simulink model "vehicle3dof"  (R2023a)
settings: Solver=FixedStepAuto  StartTime=0.0  StopTime=50  FixedStep=0.01  RelTol=1e-3
model workspace (MAT data in the model file):
  Cy_f1 = 128915.5
  Cy_r1 = 85943.6
  Izz1 = 1536.7
  a1 = 1.015
  a_max = Simulink.Parameter
  a_max.Value = [1.5 9000 9000]
  a_max.DataType = 'auto'
  a_max.Complexity = 'real'
  a_max.Dimensions = [1 3]
  a_min = Simulink.Parameter
  a_min.Value = [-1.5 -9000 -9000]
  a_min.DataType = 'auto'
  a_min.Complexity = 'real'
  a_min.Dimensions = [1 3]
  adva_max = Simulink.Parameter
  adva_max.Value = [0.05 300 300]
  adva_max.DataType = 'auto'
  adva_max.Complexity = 'real'
  adva_max.Dimensions = [1 3]
  adva_min = Simulink.Parameter
  adva_min.Value = [-0.05 -300 -300]
  adva_min.DataType = 'auto'
  adva_min.Complexity = 'real'
  adva_min.Dimensions = [1 3]
  b1 = 1.895
  done_range = Simulink.Parameter
  done_range.Value = [6 5 0.523598775598]
  done_range.DataType = 'double'
  done_range.Complexity = 'real'
  done_range.Dimensions = [1 3]
  h1 = 0.54
  noise_seed = Simulink.Parameter
  noise_seed.Value = 23341
  noise_seed.DataType = 'auto'
  noise_seed.Complexity = 'real'
  noise_seed.Dimensions = [1 1]
  punish_Q = Simulink.Parameter
  punish_Q.Value = [1 1 10 0.5]
  punish_Q.DataType = 'auto'
  punish_Q.Complexity = 'real'
  punish_Q.Dimensions = [1 4]
  punish_R = Simulink.Parameter
  punish_R.Value = [5 1e-06 1e-06]
  punish_R.DataType = 'auto'
  punish_R.Complexity = 'real'
  punish_R.Dimensions = [1 3]
  ref_A = Simulink.Parameter
  ref_A.Value = [0.3 0.8 1.5]
  ref_A.DataType = 'auto'
  ref_A.Complexity = 'real'
  ref_A.Dimensions = [1 3]
  ref_T = Simulink.Parameter
  ref_T.Value = [100 200 400]
  ref_T.DataType = 'auto'
  ref_T.Complexity = 'real'
  ref_T.Dimensions = [1 3]
  ref_V = Simulink.Parameter
  ref_V.Value = 20
  ref_V.DataType = 'auto'
  ref_V.Complexity = 'real'
  ref_V.Dimensions = [1 1]
  ref_fai = Simulink.Parameter
  ref_fai.Value = [0 0.523598775598 1.0471975512]
  ref_fai.DataType = 'auto'
  ref_fai.Complexity = 'real'
  ref_fai.Dimensions = [1 3]
  sigma_f1 = 0.1
  sigma_r1 = 0.1
  x_ini = Simulink.Parameter
  x_ini.Value = [0 0 20 0 0 0]
  x_ini.DataType = 'auto'
  x_ini.Complexity = 'real'
  x_ini.Dimensions = [1 6]
  x_max = Simulink.Parameter
  x_max.Value = [9999 9999 9999 9999 9999 9999]
  x_max.DataType = 'auto'
  x_max.Complexity = 'real'
  x_max.Dimensions = [1 6]
  x_min = Simulink.Parameter
  x_min.Value = [-9999 -9999 -9999 -9999 -9999 -9999]
  x_min.DataType = 'auto'
  x_min.Complexity = 'real'
  x_min.Dimensions = [1 6]
libraries: autolibshared x1, simulink x1
settings Model: TunableVars=a_max,a_min,adva_max,adva_min,x_ini,x_max,x_min  TunableVarsStorageClass=Auto,Auto,Auto,Auto,Auto,Auto,Auto  TunableVarsTypeQualifier=,,,,,,  ParameterArgumentNames=a_max,a_min,adva_max,adva_min,done_range,noise_seed,punish_Q,punish_R,ref_A,ref_T,ref_V,ref_fai,x_ini,x_max,x_min  Creator=hjzsj  LastModifiedBy=Asus
settings ConfigSet: Description=Config for code generation python binding.
settings SolverCC: AlgebraicLoopSolver=TrustRegion
settings OptimizationCC: DefaultParameterBehavior=Inlined  UseDivisionForNetSlopeComputation=on  UseFloatMulNetSlope=on  StrengthReduction=on  PassReuseOutputArgsAs=Individual arguments  ZeroExternalMemoryAtStartup=off  ZeroInternalMemoryAtStartup=off  NoFixptDivByZeroProtection=on  EfficientFloat2IntCast=on  OptimizeBlockOrder=speed  OptimizationPriority=Speed  OptimizationCustomize=off  MultiThreadedLoops=on  EfficientTunableParamExpr=on
settings DebuggingCC: ParameterTunabilityLossMsg=error  UnconnectedInputMsg=warning  UnconnectedOutputMsg=warning  UnconnectedLineMsg=warning  ArithmeticOperatorsInVariantConditions=warning
settings HardwareCC: ProdLongLongMode=on  TargetPreprocMaxBitsSint=64  TargetPreprocMaxBitsUint=64
settings ModelReferenceCC: EnableRefExpFcnMdlSchedulingChecks=on
settings SFSimCC: MATLABDynamicMemAlloc=off  CustomCodeUndefinedFunction=UseInterfaceOnly  SimTargetLang=C++
settings RTWCC: Description=Embedded Coder  SystemTargetFile=ert.tlc  GenCodeOnly=on  TemplateMakefile=ert_default_tmf  PostCodeGenCommand=slxpy.postprocess(modelName,buildInfo)  RetainRTWFile=on  PortableWordSizes=on  TargetLang=C++  DLArmComputeVersion=19.05
settings CodeAppCC: ForceParamTrailComments=on  CommentStyle=Multi-line  IgnoreCustomStorageClasses=off  MaxIdLength=64  OperatorAnnotations=on  SimulinkDataObjDesc=on  SFDataObjDesc=on  MATLABFcnDesc=on  MangleLength=4  InsertBlockDesc=on  StateflowObjectComments=on  MATLABSourceComments=on
settings ERTTargetCC: TargetLangStandard=C++11 (ISO)  SupportAbsoluteTime=off  CodeInterfacePackaging=C++ class  SupportComplex=off  SupportContinuousTime=on  SupportVariableSizeSignals=on  InlinedParameterPlacement=NonHierarchical  RootIOFormat=Structure reference  ERTCustomFileTemplate=example_file_process.tlc

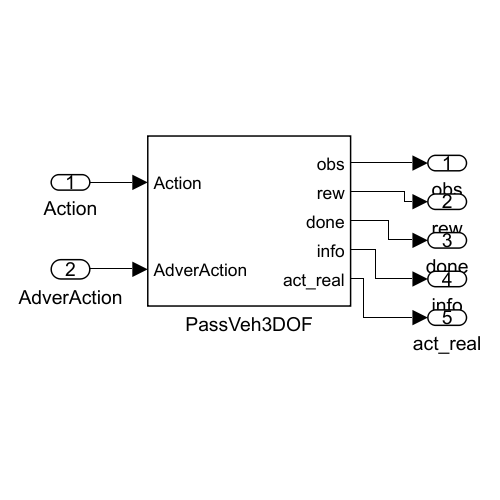
[thumbnail: Simulink's stored preview of the top-level diagram]
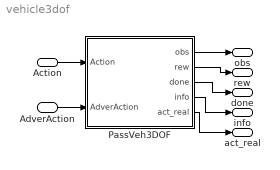
== system vehicle3dof ==
  Action : Inport  PortDimensions=3
  AdverAction : Inport  Port=2
  "PassVeh3DOF " : Subsystem
  obs : Outport
  rew : Outport  Port=2
  done : Outport  Port=3
  info : Outport  Port=4
  act_real : Outport  Port=5
  wires:
  "PassVeh3DOF "/1(obs) -> obs/1
  "PassVeh3DOF "/2(rew) -> rew/1
  Action/1 -> "PassVeh3DOF "/1(Action)
  AdverAction/1 -> "PassVeh3DOF "/2(AdverAction)
  "PassVeh3DOF "/3(done) -> done/1
  "PassVeh3DOF "/4(info) -> info/1
  "PassVeh3DOF "/5(act_real) -> act_real/1

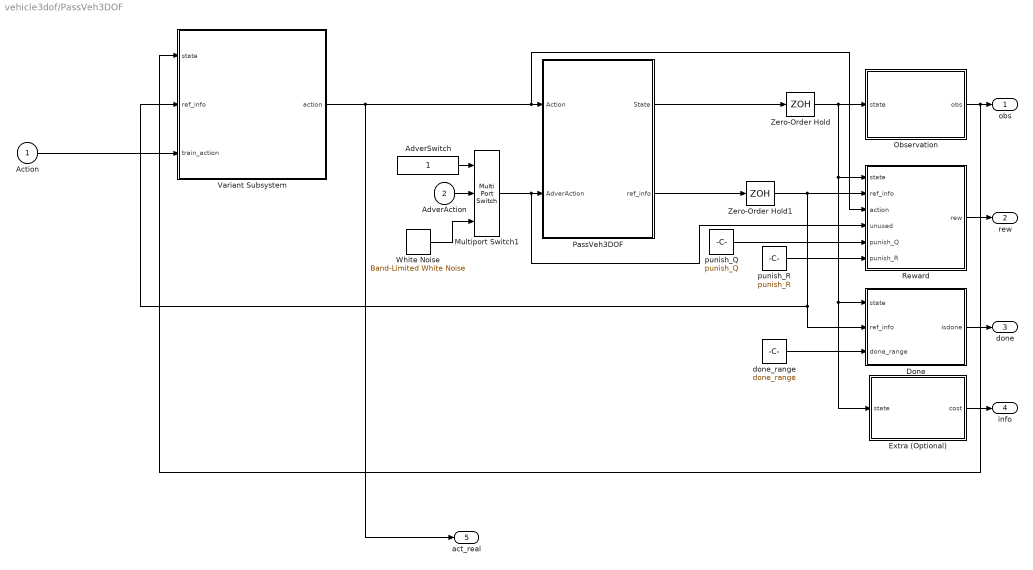
== system vehicle3dof/PassVeh3DOF  ==
  Action : Inport
  AdverAction : Inport  Port=2
  AdverSwitch : Constant
  Done : MATLAB Function  TreatAsAtomicUnit=on
  Extra (Optional) : MATLAB Function  TreatAsAtomicUnit=on
  Multiport Switch1 : MultiPortSwitch  Inputs=2  SaturateOnIntegerOverflow=off  InputSameDT=off
  Observation : MATLAB Function  TreatAsAtomicUnit=on
  "PassVeh3DOF " : Subsystem
  Reward : MATLAB Function  TreatAsAtomicUnit=on
  Variant Subsystem : Subsystem  Variant=on  VariantControlMode=label  LabelModeActiveChoice=Train
  White Noise : simulink/Sources/Band-Limited White Noise  Cov=[0.5, 100, 100]  Ts=0.02  seed=noise_seed
  Zero-Order Hold : ZeroOrderHold  SampleTime=-1
  Zero-Order Hold1 : ZeroOrderHold  SampleTime=-1
  done_range : Constant  Value=done_range
  punish_Q : Constant  Value=punish_Q
  punish_R : Constant  Value=punish_R
  obs : Outport
  rew : Outport  Port=2
  done : Outport  Port=3
  info : Outport  Port=4
  act_real : Outport  Port=5
  wires:
  Action/1 -> Variant Subsystem/3(train_action)
  Multiport Switch1/1 -> Reward/4(unused), "PassVeh3DOF "/2(AdverAction)
  AdverSwitch/1 -> Multiport Switch1/1
  White Noise/1 -> Multiport Switch1/3
  AdverAction/1 -> Multiport Switch1/2
  Zero-Order Hold/1 -> Extra (Optional)/1(state), Done/1(state), Reward/1(state), Observation/1(state)
  "PassVeh3DOF "/1(State) -> Zero-Order Hold/1
  Observation/1(obs) -> Variant Subsystem/1(state), obs/1
  Reward/1(rew) -> rew/1
  Extra (Optional)/1(cost) -> info/1
  "PassVeh3DOF "/2(ref_info) -> Zero-Order Hold1/1
  punish_Q/1 -> Reward/5(punish_Q)
  punish_R/1 -> Reward/6(punish_R)
  done_range/1 -> Done/3(done_range)
  Done/1(isdone) -> done/1
  Zero-Order Hold1/1 -> Done/2(ref_info), Variant Subsystem/2(ref_info), Reward/2(ref_info)
  Variant Subsystem/1(action) -> Reward/3(action), "PassVeh3DOF "/1("Action "), act_real/1

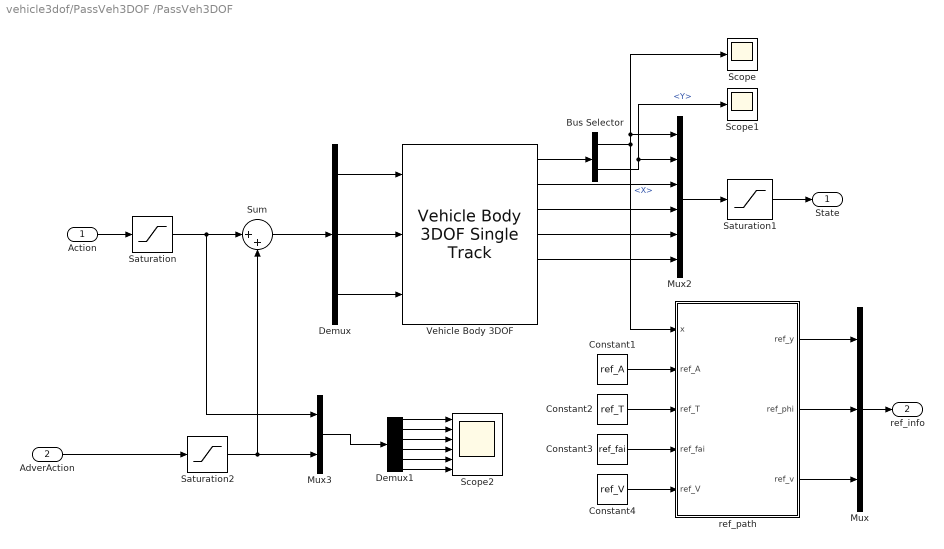
== system vehicle3dof/PassVeh3DOF /PassVeh3DOF  ==
  "Action " : Inport
  AdverAction : Inport  Port=2
  " ref_path " : MATLAB Function  TreatAsAtomicUnit=on
  Bus Selector : BusSelector  OutputSignals=InertFrm.Cg.Disp.X,InertFrm.Cg.Disp.Y
  Constant1 : Constant  Value=ref_A
  Constant2 : Constant  Value=ref_T
  Constant3 : Constant  Value=ref_fai
  Constant4 : Constant  Value=ref_V
  Demux : Demux  Outputs=3
  Demux1 : Demux  Outputs=6
  Mux : Mux  Inputs=3
  Mux2 : Mux  Inputs=6
  Mux3 : Mux  Inputs=2
  Saturation : Saturate  UpperLimit=a_max  LowerLimit=a_min
  Saturation1 : Saturate  UpperLimit=x_max  LowerLimit=x_min
  Saturation2 : Saturate  UpperLimit=adva_max  LowerLimit=adva_min
  Scope : Scope
  Scope1 : Scope
  Scope2 : Scope  NumInputPorts=6
  Sum : Sum  Inputs=|++
  "Vehicle Body 3DOF " : autolibshared/Vehicle Body 3DOF Single Track  trackMode=Single (bicycle)  inputMode=External longitudinal forces  frontSteerMode=on  rearSteerMode=off  windMode=off  muMode=off  extFMode=off  extMMode=off  htchFMode=off  htchMMode=off  extXo=off  extpsio=off  extxdoto=off  extro=off  extYo=off  extTamb=off  extydoto=off  aMode=2  NF=2  NR=2  m=1470  a=a1  b=b1  h=h1  dh=1  hh=0.2  X_o=x_ini(1)  xdot_o=x_ini(3)  CalphaMode=off  sigmaMode=on  d=0  hl=0  w=[1.4,1.4]  Cy_f=Cy_f1  Cy_r=Cy_r1  sigma_f=sigma_f1  sigma_r=sigma_r1  alpha_f_brk=[-.1 .1]  Cy_f_data=[-9e3 9e3]  alpha_r_brk=[-.1 .1]  Cy_r_data=[-9e3 9e3]  Y_o=x_ini(2)  ydot_o=x_ini(4)  Izz=Izz1  psi_o=x_ini(5)  r_o=x_ini(6)  Af=2.2  Cd=.3  Cl=.18  Cpm=-0.15  beta_w=[0:0.01:0.3]  Cs=[0:0.03:0.9]  Cym=[0:0.01:0.3]  Pabs=101325  Tair=273  g=9.81  mu=1  xdot_tol=.01  Fznom=5000  Fxtire_sat=7e4  Fytire_sat=7e4  longOff=0  latOff=0  vertOff=0  wrapAng=off
  State : Outport  VectorParamsAs1DForOutWhenUnconnected=off
  ref_info : Outport  Port=2  VectorParamsAs1DForOutWhenUnconnected=off
  wires:
  Mux2/1 -> Saturation1/1
  "Action "/1 -> Saturation/1
  Saturation1/1 -> State/1
  Saturation/1 -> Sum/1, Mux3/1
  Demux/1 -> "Vehicle Body 3DOF "/1
  Demux/2 -> "Vehicle Body 3DOF "/2
  "Vehicle Body 3DOF "/1 -> Bus Selector/1
  Bus Selector/1 -> " ref_path "/1(x), Scope/1, Mux2/1  "<X>"
  Bus Selector/2 -> Scope1/1, Mux2/2  "<Y>"
  "Vehicle Body 3DOF "/2 -> Mux2/3
  "Vehicle Body 3DOF "/3 -> Mux2/4
  "Vehicle Body 3DOF "/4 -> Mux2/5
  "Vehicle Body 3DOF "/5 -> Mux2/6
  Demux/3 -> "Vehicle Body 3DOF "/3
  Mux3/1 -> Demux1/1
  Saturation2/1 -> Sum/2, Mux3/2
  Sum/1 -> Demux/1
  Constant4/1 -> " ref_path "/5(ref_V)
  Constant2/1 -> " ref_path "/3(ref_T)
  " ref_path "/2(ref_phi) -> Mux/2
  Constant1/1 -> " ref_path "/2(ref_A)
  " ref_path "/1(ref_y) -> Mux/1
  " ref_path "/3(ref_v) -> Mux/3
  Constant3/1 -> " ref_path "/4(ref_fai)
  Mux/1 -> ref_info/1
  Demux1/1 -> Scope2/1
  Demux1/2 -> Scope2/2
  Demux1/3 -> Scope2/3
  Demux1/4 -> Scope2/4
  Demux1/5 -> Scope2/5
  Demux1/6 -> Scope2/6
  AdverAction/1 -> Saturation2/1

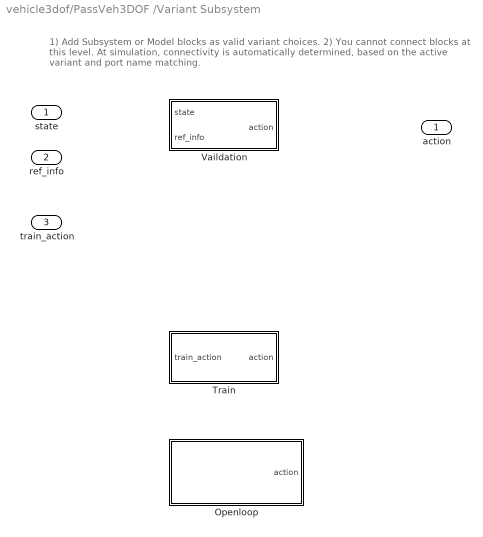
== system vehicle3dof/PassVeh3DOF /Variant Subsystem ==
  note: 1) Add Subsystem or Model blocks as valid variant choices.
      | 2) You cannot connect blocks at this level. At simulation, connectivity is automatically
      | determined, based on the active variant and port name matching.
  state : Inport
  ref_info : Inport  Port=2
  train_action : Inport  Port=3
  Openloop : Subsystem  VariantControl=Opneloop
  Train : Subsystem  VariantControl=Train
  Vaildation : Subsystem  VariantControl=Validation
  action : Outport

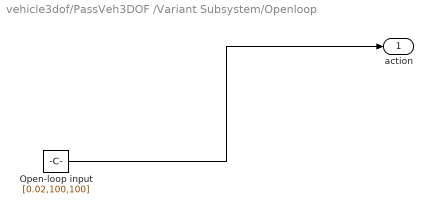
== system vehicle3dof/PassVeh3DOF /Variant Subsystem/Openloop ==
  Open-loop input : Constant  Value=[0.02,100,100]
  action : Outport
  wires:
  Open-loop input/1 -> action/1

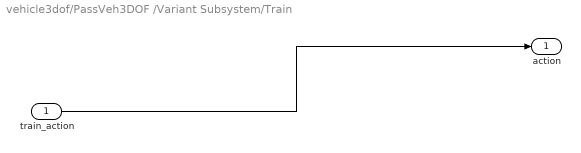
== system vehicle3dof/PassVeh3DOF /Variant Subsystem/Train ==
  train_action : Inport
  action : Outport
  wires:
  train_action/1 -> action/1

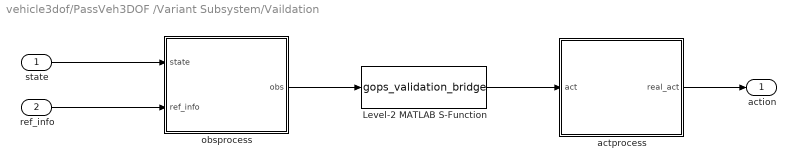
== system vehicle3dof/PassVeh3DOF /Variant Subsystem/Vaildation ==
  state : Inport
  ref_info : Inport  Port=2
  Level-2 MATLAB S-Function : M-S-Function  FunctionName=gops_validation_bridge  Parameters='E:\PHD\Project\GOPS\repov38\paper_results\apprfunc\model.pt'
  actprocess : MATLAB Function  TreatAsAtomicUnit=on
  obsprocess : MATLAB Function  TreatAsAtomicUnit=on
  action : Outport
  wires:
  obsprocess/1(obs) -> Level-2 MATLAB S-Function/1
  Level-2 MATLAB S-Function/1 -> actprocess/1(act)
  state/1 -> obsprocess/1(state)
  ref_info/1 -> obsprocess/2(ref_info)
  actprocess/1(real_act) -> action/1

== matlab function vehicle3dof/PassVeh3DOF /Done ==
  data: state input; isdone output; ref_info input; done_range input
function isdone = fun_done(state, ref_info, done_range)
false = abs(state(2)-ref_info(1))>done_range(1) ...
        || abs(state(3)-ref_info(3))>done_range(2) ...
        || abs(state(5)-ref_info(2))>done_range(3);
isdone = false;

== matlab function vehicle3dof/PassVeh3DOF /Variant Subsystem/Vaildation/obsprocess ==
  data: state input; obs output; ref_info input
function obs = fun_done(state, ref_info)
    ref_A = [0.3, 0.8, 1.5];
    ref_T = [100, 200, 400];
    ref_fai= [0, pi/ 6, pi/3];
    delta_t = 0.01;
    ref_v = ref_info(3);
    obs = zeros(6,1);
    obs(1) = state(1)*0.001;
    obs(2) = state(2) -ref_info(1);
    obs(3) = state(3) -ref_info(3);
    obs(4) = state(4);
    obs(5) = (state(5)- ref_info(2))*2.4;
    obs(6) = state(6)*2;
%     for t=7:1:27
%         x = state(1) + delta_t*ref_v*(t-6);
%         obs(t) = ref_A(1)*sin(2*pi/ref_T(1)*x + ref_fai(1)) + ref_A(2)*sin(2*pi/ref_T(2)*x + ref_fai(2)) + ref_A(3)*sin(2*pi/ref_T(3)*x + ref_fai(3));
%     end

end

== matlab function vehicle3dof/PassVeh3DOF /Variant Subsystem/Vaildation/actprocess ==
  data: act input; real_act output
function real_act = fun_act(act)
real_act =act;
real_act(1) = act(1)/10;
real_act(2) = act(2)*1000;
real_act(3) = act(3)*1000;
end

== matlab function vehicle3dof/PassVeh3DOF /Extra (Optional) ==
  data: state input; cost output
function cost = fun_extra(state)
cost = 0;

== matlab function vehicle3dof/PassVeh3DOF /Observation ==
  data: state input; obs output
function obs = fun_obs(state)
obs = state;

== matlab function vehicle3dof/PassVeh3DOF /Reward ==
  data: state input; ref_info input; rew output; action input; unused input; punish_Q input; punish_R input
function rew = fun_rew(state, ref_info, action, ~,  punish_Q, punish_R)
rew = punish_Q(1)*(state(2)-ref_info(1))^2 + punish_Q(2)*(state(3)-ref_info(3))^2 ...
    + punish_Q(3)*(state(5)-ref_info(2))^2 + punish_Q(4)*state(6)^2 ...
    + punish_R(1)*(action(1))^2 + punish_R(2)*(action(2))^2 + punish_R(3)*(action(3))^2;
rew = -rew;

== matlab function vehicle3dof/PassVeh3DOF /PassVeh3DOF / ref_path  ==
  data: x input; ref_y output; ref_phi output; ref_v output; ref_A input; ref_T input; ref_fai input; ref_V input
function [ref_y, ref_phi, ref_v]= fcn(x, ref_A, ref_T, ref_fai, ref_V)
ref_y = ref_A(1)*sin(2*pi/ref_T(1)*x + ref_fai(1)) + ref_A(2)*sin(2*pi/ref_T(2)*x + ref_fai(2)) + ref_A(3)*sin(2*pi/ref_T(3)*x + ref_fai(3));
ref_phi_k = ref_A(1)*2*pi/ref_T(1)*cos(2*pi/ref_T(1)*x + ref_fai(1)) + ref_A(2)*2*pi/ref_T(2)*cos(2*pi/ref_T(2)*x + ref_fai(2)) + ref_A(3)*2*pi/ref_T(3)*cos(2*pi/ref_T(3)*x + ref_fai(3));
ref_phi = atan(ref_phi_k);
ref_v = ref_V;
